simulink model "MotorPlant_XY"  (R2016b)
settings: Solver=VariableStepAuto  StartTime=0.0  StopTime=20  RelTol=1e-3
InitFcn:
  | Km = 0.01; %Toque constant
  | Kb = 0.01; %Back-emf constant
  | Jm = 0.01; %Rotor inertia
  | F = 0.1; %Rotor damping
  | Ra = 1; %Armature resistance
  | La = 0.5; %Armature inductance
values from neighbouring files (symbols this model uses):
  K = acker(A_D,B_D,p)    [linearization_and_Controller.m]
  Ts = 0.01    [linearization_and_Controller.m]
libraries: simulink x4
settings Model: Creator=Alire  LastModifiedBy=ProBook
settings SFSimCC: SimUseLocalCustomCode=on
settings RTWCC: RTWUseLocalCustomCode=on

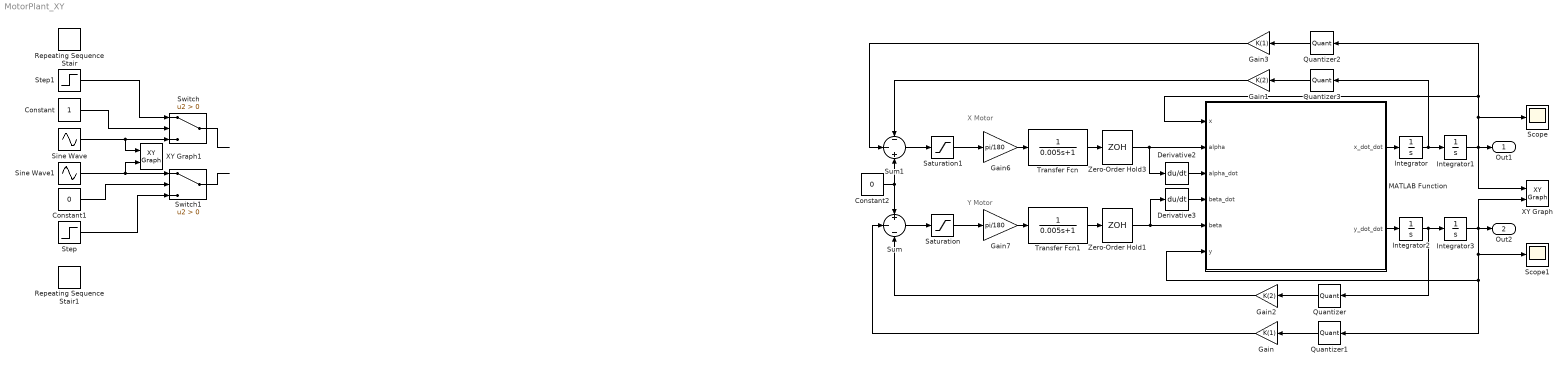
== system MotorPlant_XY ==
  note: X Motor
  note: Y Motor
  Constant : Constant
  Constant1 : Constant  Value=0
  Constant2 : Constant  Value=0
  Derivative2 : Derivative
  Derivative3 : Derivative
  Gain : Gain  Gain=K(1)
  Gain1 : Gain  Gain=K(2)
  Gain2 : Gain  Gain=K(2)
  Gain3 : Gain  Gain=K(1)
  Gain6 : Gain  Gain=pi/180
  Gain7 : Gain  Gain=pi/180
  Integrator : Integrator
  Integrator1 : Integrator  InitialCondition=0.1
  Integrator2 : Integrator
  Integrator3 : Integrator  InitialCondition=-0.1
  MATLAB Function : MATLAB Function  TreatAsAtomicUnit=on
  Quantizer{,1..3} (4 alike) : Quantizer  QuantizationInterval=Ts
  Repeating Sequence Stair : simulink/Sources/Repeating Sequence Stair  OutValues=[0.07 -0.07 -0.07 0.07]  tsamp=10  OutMin=[]  OutMax=[]  OutDataTypeStr=double  OutputDataTypeScalingMode=double  OutDataType=fixdt(0,8)  ConRadixGroup=Best Precision: Vector-wise  OutScaling=2^-12
  Repeating Sequence Stair1 : simulink/Sources/Repeating Sequence Stair  OutValues=[0.8 0.8 -0.8 -0.8]  tsamp=10  OutMin=[]  OutMax=[]  OutDataTypeStr=double  OutputDataTypeScalingMode=double  OutDataType=fixdt(0,8)  ConRadixGroup=Best Precision: Vector-wise  OutScaling=2^-12
  Saturation : Saturate  UpperLimit=+5  LowerLimit=-5
  Saturation1 : Saturate  UpperLimit=+5  LowerLimit=-5
  Scope : Scope
  Scope1 : Scope
  Sine Wave : Sin  Amplitude=0.07  Frequency=0.1  SampleTime=Ts
  Sine Wave1 : Sin  Amplitude=0.07  Frequency=0.1  Phase=+pi/2  SampleTime=Ts
  Step : Step  Time=0  After=0  SampleTime=0.02
  Step1 : Step  Time=0  After=0  SampleTime=0.02
  Sum : Sum  Inputs=+|-|-
  Sum1 : Sum  Inputs=-|-|+
  Switch : Switch  Criteria=u2 > Threshold
  Switch1 : Switch  Criteria=u2 > Threshold
  Transfer Fcn : TransferFcn  Denominator=[0.005 1]
  Transfer Fcn1 : TransferFcn  Denominator=[0.005 1]
  XY Graph : simulink/Sinks/XY Graph  xmin=-0.2  xmax=0.2  ymin=-0.2  ymax=0.2  st=-1
  XY Graph1 : simulink/Sinks/XY Graph  xmin=-0.2  xmax=0.2  ymin=-0.2  ymax=0.2  st=-1
  Zero-Order Hold1 : ZeroOrderHold  SampleTime=Ts
  Zero-Order Hold3 : ZeroOrderHold  SampleTime=Ts
  Out1 : Outport  SignalName=X
  Out2 : Outport  Port=2  SignalName=Y
  wires:
  Quantizer/1 -> Gain2/1
  Quantizer1/1 -> Gain/1
  Integrator2/1 -> Integrator3/1, Quantizer/1
  Integrator1/1 -> XY Graph/1, Out1/1, Scope/1, Quantizer2/1, MATLAB Function/1(x)
  Quantizer3/1 -> Gain1/1
  Quantizer2/1 -> Gain3/1
  Sum/1 -> Saturation/1
  Gain2/1 -> Sum/3
  Gain/1 -> Sum/2
  Constant2/1 -> Sum1/3, Sum/1
  Sum1/1 -> Saturation1/1
  Gain1/1 -> Sum1/1
  Gain3/1 -> Sum1/2
  Derivative3/1 -> MATLAB Function/4(beta_dot)
  Derivative2/1 -> MATLAB Function/3(alpha_dot)
  Integrator/1 -> Integrator1/1, Quantizer3/1
  MATLAB Function/2(y_dot_dot) -> Integrator2/1
  MATLAB Function/1(x_dot_dot) -> Integrator/1
  Transfer Fcn/1 -> Zero-Order Hold3/1
  Gain6/1 -> Transfer Fcn/1
  Zero-Order Hold3/1 -> Derivative2/1, MATLAB Function/2(alpha)
  Saturation1/1 -> Gain6/1
  Gain7/1 -> Transfer Fcn1/1
  Transfer Fcn1/1 -> Zero-Order Hold1/1
  Saturation/1 -> Gain7/1
  Zero-Order Hold1/1 -> Derivative3/1, MATLAB Function/5(beta)
  Integrator3/1 -> XY Graph/2, Out2/1, MATLAB Function/6(y), Quantizer1/1, Scope1/1
  Step/1 -> Switch1/3
  Switch1/1 -> ?
  Sine Wave1/1 -> XY Graph1/2, Switch1/1
  Constant1/1 -> Switch1/2
  Switch/1 -> ?
  Step1/1 -> Switch/1
  Constant/1 -> Switch/2
  Sine Wave/1 -> XY Graph1/1, Switch/3

== matlab function MotorPlant_XY/MATLAB Function ==
  data: x input; alpha input; x_dot_dot output; alpha_dot input; beta_dot input; beta input; y input; y_dot_dot output
function [x_dot_dot,y_dot_dot] = fcn(x,alpha,alpha_dot,beta_dot,beta,y)
g = 9.81;
B = 5/7;
x_dot_dot = (B)*(x*(alpha_dot^2)+y*alpha_dot*beta_dot) - (B)*g*sin(alpha);
y_dot_dot = (B)*(y*(beta_dot^2)+x*alpha_dot*beta_dot)- (B)*g*sin(beta);
